simulink model "DC_Motor_Velocity"  (R2018a)
settings: Solver=VariableStepAuto  StartTime=0.0  StopTime=10  RelTol=1e-3
libraries: simulink x2
settings Model: Creator=barak  LastModifiedBy=barak

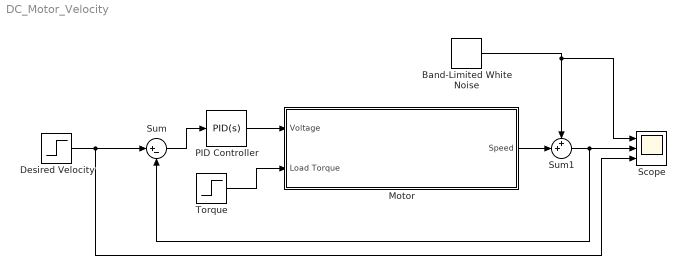
== system DC_Motor_Velocity ==
  Band-Limited White Noise : simulink/Sources/Band-Limited White Noise  Cov=[0.1]  Ts=1  seed=[0]
  Desired Velocity : Step  SampleTime=0
  Motor : Subsystem
  PID Controller : simulink/Continuous/PID Controller  Controller=PID  TimeDomain=Continuous-time  SampleTime=-1  IntegratorMethod=Forward Euler  FilterMethod=Forward Euler  Form=Parallel  UseFilter=on  ControllerParametersSource=internal  P=2.65591901691588  I=50.6808089955632  D=-0.000116199422511301  N=22856.5595208321  InitialConditionSource=internal  InitialConditionForIntegrator=0  InitialConditionForFilter=0  ExternalReset=none  LimitOutput=off  UpperSaturationLimit=inf  LowerSaturationLimit=-inf  LinearizeAsGain=on  AntiWindupMode=none  Kb=1  TrackingMode=off  Kt=1  PParamMin=[]  PParamMax=[]  IParamMin=[]  IParamMax=[]  DParamMin=[]  DParamMax=[]  NParamMin=[]  NParamMax=[]  KbParamMin=[]  KbParamMax=[]  KtParamMin=[]  KtParamMax=[]  POutMin=[]  POutMax=[]  IOutMin=[]  IOutMax=[]  DOutMin=[]  DOutMax=[]  NOutMin=[]  NOutMax=[]  KbOutMin=[]  KbOutMax=[]  KtOutMin=[]  KtOutMax=[]  IntegratorOutMin=[]  IntegratorOutMax=[]  FilterOutMin=[]  FilterOutMax=[]  SumOutMin=[]  SumOutMax=[]  SumI1OutMin=[]  SumI1OutMax=[]  SumI2OutMin=[]  SumI2OutMax=[]  SumI3OutMin=[]  SumI3OutMax=[]  SumDOutMin=[]  SumDOutMax=[]  SaturationOutMin=[]  SaturationOutMax=[]  IntegratorContinuousStateAttributes=''  IntegratorStateMustResolveToSignalObject=off  IntegratorRTWStateStorageClass=Auto  FilterContinuousStateAttributes=''  FilterStateMustResolveToSignalObject=off  FilterRTWStateStorageClass=Auto  DifferentiatorICPrevScaledInput=0  DifferentiatorOutMin=[]  DifferentiatorOutMax=[]  FilterDiffOutCoefMin=[]  FilterDiffOutCoefMax=[]  SumDenOutMin=[]  SumDenOutMax=[]  SumNumOutMin=[]  SumNumOutMax=[]  ReciprocalOutMin=[]  ReciprocalOutMax=[]  DivideOutMin=[]  DivideOutMax=[]  TunerSelectOption=Transfer Function Based (PID Tuner App)
  Scope : Scope  NumInputPorts=3
  Sum : Sum  Inputs=|+-
  Sum1 : Sum  Inputs=++|
  "Torque " : Step  Time=20  After=0  SampleTime=0
  wires:
  PID Controller/1 -> Motor/1(Voltage)
  Sum/1 -> PID Controller/1
  Desired Velocity/1 -> Scope/3, Sum/1
  "Torque "/1 -> Motor/2("Load Torque ")
  Band-Limited White Noise/1 -> Scope/1, Sum1/1
  Motor/1("Speed ") -> Sum1/2
  Sum1/1 -> Scope/2, Sum/2

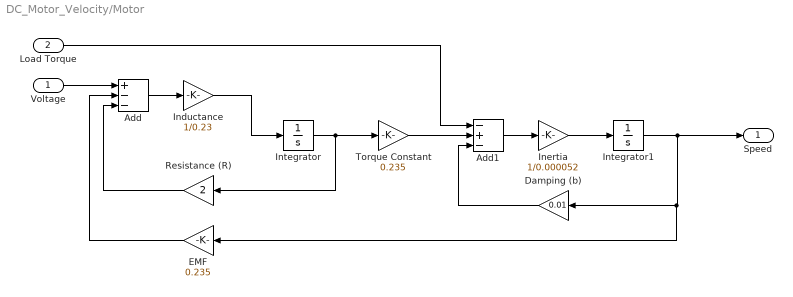
== system DC_Motor_Velocity/Motor ==
  Voltage : Inport
  "Load Torque " : Inport  Port=2
  Add : Sum  Inputs=+--
  Add1 : Sum  Inputs=-+-
  Damping (b) : Gain  Gain=0.01
  EMF : Gain  Gain=0.235
  Inductance : Gain  Gain=1/0.23
  "Inertia " : Gain  Gain=1/0.000052
  Integrator : Integrator
  Integrator1 : Integrator
  Resistance (R) : Gain  Gain=2
  Torque Constant : Gain  Gain=0.235
  "Speed " : Outport
  wires:
  Voltage/1 -> Add/1
  Add/1 -> Inductance/1
  Inductance/1 -> Integrator/1
  Integrator/1 -> Resistance (R)/1, Torque Constant/1
  Resistance (R)/1 -> Add/3
  Add1/1 -> "Inertia "/1
  "Inertia "/1 -> Integrator1/1
  Integrator1/1 -> EMF/1, Damping (b)/1, "Speed "/1
  EMF/1 -> Add/2
  "Load Torque "/1 -> Add1/1
  Torque Constant/1 -> Add1/2
  Damping (b)/1 -> Add1/3
